simulink model "Model_Linearisierung_final"  (R2023b)
settings: Solver=FixedStepAuto  StartTime=0.0  StopTime=Inf  FixedStep=1e-4  RelTol=1e-3
PostLoadFcn:
  | if any(exist('dsrtsu_mdlpostloadfcn', 'file') ~= 0), dsrtsu_mdlpostloadfcn('Execute', bdroot); end
InitFcn:
  | , if any(exist('rtifpga_mdlclblib', 'file') ~= 0), rtifpga_mdlclblib('Init', bdroot); end,
  | , if any(exist('dsmpb_private', 'file') ~= 0), dsmpb_private('dsmpb_mdlclblib', 'Init', bdroot); end,
  | load('LUT_BRUSA_jax_grad.mat')
  | load('daten_nichtlinear_interpoliert.mat')
  | load('Maschinendaten.mat')
values from neighbouring files (symbols this model uses):
  delta_id = id_fine(2)-id_fine(1)    [Messdaten_Interpoliert.m]    (also in daten_nichtlinear_interpoliert.mat = 2.52525252525)
  delta_iq = iq_fine(2)-iq_fine(1)    [Messdaten_Interpoliert.m]    (also in daten_nichtlinear_interpoliert.mat = 5.05050505051)
  I_max = 170    [Maschinendaten.mat]    (also in Maschinendaten_Vorgabe.m; test_ModelParameters.m = evalin('base', 'I_max'); test_StrategySelection.m = tc.readConstant(tc.BLK_Imax))
  ID = [-250 -250 -250 -250 -250 -250 -250 -250 -250 -250 -250 -250 ... (10000 elements, 100x100)]    [daten_nichtlinear_interpoliert.mat]
  id_fine = linspace(min(id_vec), max(id_vec), 100)    [Messdaten_Interpoliert.m]    (also in daten_nichtlinear_interpoliert.mat = [-250 -247.474747475 -244.949494949 -242.424242424 -239.8989)
  IQ = [-250 -244.949494949 -239.898989899 -234.848484848 -229.797979798 -224.747474747 -219.696969697 -214.646464646 -209.595959596 -204.545454545 -199.494949495 -194.444444444 ... (10000 elements, 100x100)]    [daten_nichtlinear_interpoliert.mat]
  iq_fine = linspace(min(iq_vec), max(iq_vec), 100)    [Messdaten_Interpoliert.m]    (also in daten_nichtlinear_interpoliert.mat = [-250 -244.949494949 -239.898989899 -234.848484848 -229.7979)
  Ldd = Ldd_fine    [Messdaten_Interpoliert.m]    (also in daten_nichtlinear_interpoliert.mat = [0.000225276031415 0.000225750625371 0.000226241749969 0.000)
  Ldq = Ldq_fine    [Messdaten_Interpoliert.m]    (also in daten_nichtlinear_interpoliert.mat = [1.31113456519e-05 1.34236782585e-05 1.31001168558e-05 1.236)
  Lqd = Lqd_fine    [Messdaten_Interpoliert.m]    (also in daten_nichtlinear_interpoliert.mat = [7.22855329514e-05 7.00325573553e-05 6.7613098921e-05 6.5016)
  Lqq = Lqq_fine    [Messdaten_Interpoliert.m]    (also in daten_nichtlinear_interpoliert.mat = [0.000286039721686 0.000286453471045 0.000286025480511 0.000)
  n_max = 11000    [Maschinendaten.mat]    (also in Maschinendaten_Vorgabe.m; test_ModelParameters.m = evalin('base', 'n_max'); test_StrategySelection.m = tc.readConstant(tc.BLK_nmax))
  p = 3    [Maschinendaten.mat]    (also in Maschinendaten_Vorgabe.m; Messdaten_Interpoliert.m; test_ModelParameters.m = evalin('base', 'p'))
  Psid = Psid_fine    [Messdaten_Interpoliert.m]    (also in daten_nichtlinear_interpoliert.mat = [0.00602681114795 0.00609490588107 0.00615917040906 0.006219)
  Psiq = Psiq_fine    [Messdaten_Interpoliert.m]    (also in daten_nichtlinear_interpoliert.mat = [-0.166252688687 -0.164805403122 -0.163363500753 -0.16192610)
  Rs = 0.018    [Maschinendaten.mat]    (also in Maschinendaten_Vorgabe.m; test_ModelParameters.m = evalin('base', 'Rs'))
  U_dc = 560    [Maschinendaten.mat]    (also in Maschinendaten_Vorgabe.m; test_ModelParameters.m = evalin('base', 'U_dc'))
  U_max = 323.316150746    [Maschinendaten.mat]    (also in Maschinendaten_Vorgabe.m = U_dc / sqrt(3); test_ModelParameters.m = evalin('base', 'U_max'))
(part 1 of 3)
PreSaveFcn:
  | , if any(exist('dsmpb_private', 'file') ~= 0), dsmpb_private('dsmpb_mdlclblib', 'PreSave', bdroot); end,
CloseFcn:
  | , if any(exist('dsmpb_private', 'file') ~= 0), dsmpb_private('dsmpb_mdlclblib', 'Close', bdroot); end,
settings Model: DSRTSU_INTERNAL_RTIFPGA=210  DSRTSU_INTERNAL_RTISTBM_VER=24.2  DSMPB_ID_DATA={'1013',struct('BlockId','890db5c5-f774-4909-8d7b-80034ce0aceb','SignalIds',{{'dc619e18-1e49-4960-b686-3641b5b4e79b'}}),'722',struct('BlockId','8930e04f-7b9c-444e-9dfc-cdc89f8efc2c','SignalIds',{{'dce83508-d3d2-4435-9767-da790707202b'}}),'723',struct('BlockId','5d03b730-b193-419a-83cc-f730a6167e44','SignalIds',{{'20e4a8f8-d10b-4aad-9fba-86ba3280d00f'}}),'724',struct('BlockId','af5ca0db-6ef4-4fd1-9517-7edab6eec934','SignalIds',{{'0119e9a3-0335-4eef-8de2-1e0c5afd4a30'}})}  Creator=Student  LastModifiedBy=sarah
settings OptimizationCC: BlockReduction=off  ConditionallyExecuteInputs=off  OptimizeBlockIOStorage=off  BufferReuse=off
settings DebuggingCC: TasksWithSamePriorityMsg=none
settings HardwareCC: ProdBitPerLong=64  ProdLargestAtomicInteger=Integer  ProdWordSize=32  ProdLongLongMode=on  ProdHWDeviceType=Custom Processor->Custom
settings ModelReferenceCC: EnableParallelModelReferenceBuilds=on
settings RTWCC: Description=dSPACE Target DSRT - Generates SIC files for import by ConfigurationDesk and VEOS. Provides code generation for Simulink models imported in ConfigurationDesk.  SystemTargetFile=dsrt.tlc  GenCodeOnly=on  MakeCommand=make_dsrt  TemplateMakefile=dsrt_default_tmf  RTWVerbose=off
settings STFCustomTargetCC: ParMdlRefBuildCompliant=on  SystemTargetFile=dsrt.tlc
settings GRTTargetCC: CompOptLevelCompliant=off  ConcurrentExecutionCompliant=off  CombineOutputUpdateFcns=off  MatFileLogging=off  CPPClassGenCompliant=off  UseToolchainInfoCompliant=off

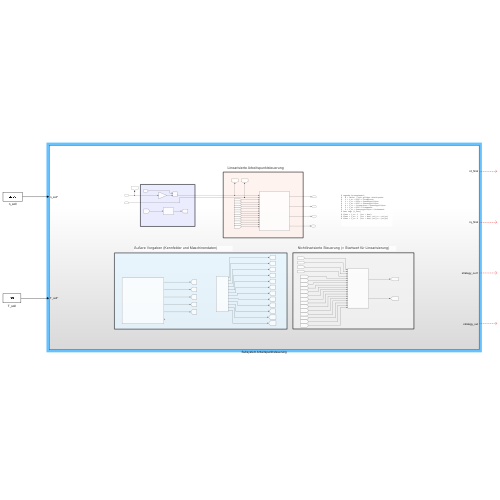
[thumbnail: Simulink's stored preview of the top-level diagram]
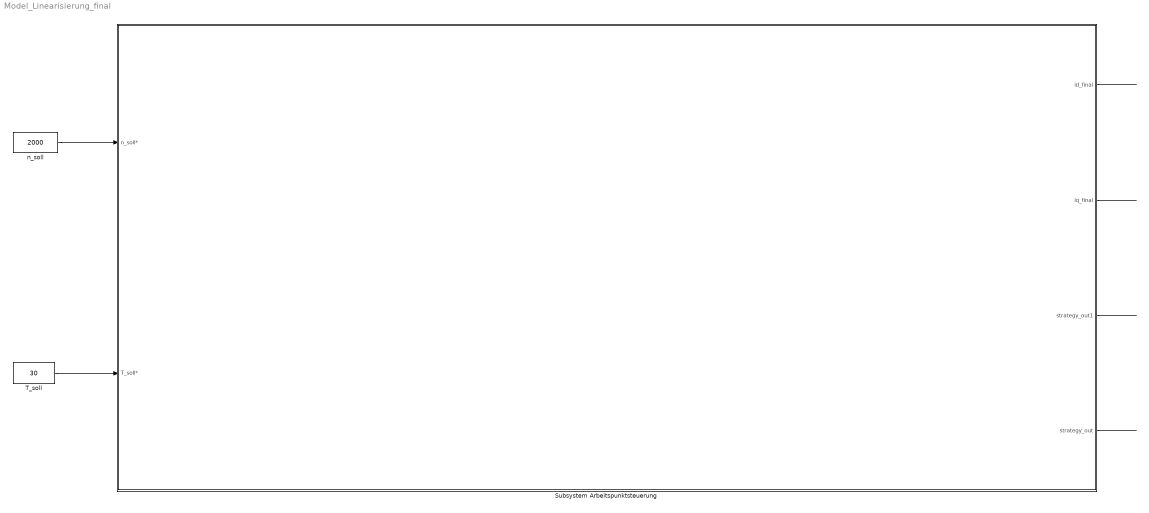
== system Model_Linearisierung_final ==
  Subsystem Arbeitspunktsteuerung : Subsystem
  T_soll : Constant  Value=30
  n_soll : Constant  Value=2000
  wires:
  n_soll/1 -> Subsystem Arbeitspunktsteuerung/1(n_soll*)
  T_soll/1 -> Subsystem Arbeitspunktsteuerung/2(T_soll*)
  Subsystem Arbeitspunktsteuerung/1(id_final) -> ?
  Subsystem Arbeitspunktsteuerung/2(iq_final) -> ?
  Subsystem Arbeitspunktsteuerung/4(strategy_out) -> ?
  Subsystem Arbeitspunktsteuerung/3(strategy_out1) -> ?

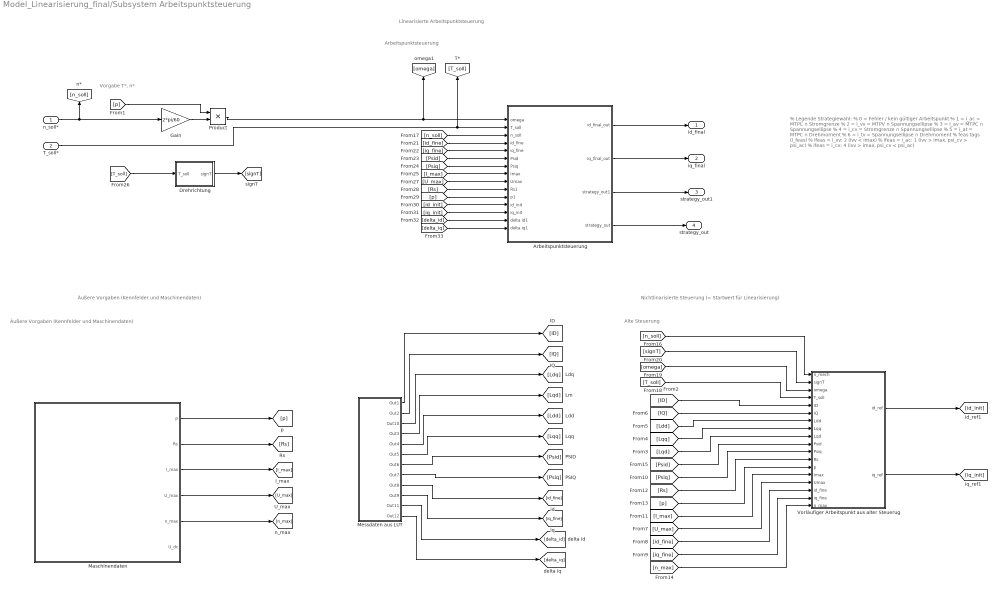
== system Model_Linearisierung_final/Subsystem Arbeitspunktsteuerung ==
  note: Vorgabe T*, n*
  note: % Legende Strategiewahl:
      | % 0 = Fehler / kein gültiger Arbeitspunkt
      | % 1 = i_ac = MTPC ∩ Stromgrenze
      | % 2 = i_vv = MTPV ∩ Spannungsellipse
      | % 3 = i_av = MTPC ∩ Spannungsellipse
      | % 4 = i_cv = Stromgrenze ∩ Spannungsellipse
      | % 5 = i_at = MTPC ∩ Drehmoment
      | % 6 = i_tv = Spannungsellipse ∩ Drehmoment
      | % feas tags (i_feas)
      | % ifeas = i_vv: 2 (ivv < imax)
      | % ifeas = i_ac: 1 (ivv > imax, psi_cv > psi_ac)
      | % ifeas = i_cv: 4 (ivv > imax, psi_cv < psi_ac)
  note: Nichtlinarisierte Steuerung (= Startwert für Linearisierung)
  note: Äußere Vorgaben (Kennfelder und Maschinendaten)
  note: Alte Steuerung
  note: Äußere Vorgaben (Kennfelder und Maschinendaten)
  note: Arbeitspunktsteuerung
  note: Linearisierte Arbeitspunktsteuerung
  n_soll* : Inport
  T_soll* : Inport  Port=2
  Arbeitspunktsteuerung : Subsystem
  Drehrichtung : MATLAB Function  Tag=<DSModel=2_'Model_Sarah'>  TreatAsAtomicUnit=on
      settings: AttributesFormatString=<DSModel='Model_Sarah'>
  Gain : Gain  Gain=2*pi/60
  Maschinendaten : Subsystem  Tag=<DSModel=5_'Model_Sarah'>
      settings: AttributesFormatString=<DSModel='Model_Sarah'>
  Messdaten aus LUT : Subsystem  Tag=<DSModel=4_'Model_Sarah'>
      settings: AttributesFormatString=<DSModel='Model_Sarah'>
  Product : Product
  Vorläufiger Arbeitspunkt aus alter Steuerug : Subsystem
  id_final : Outport
  iq_final : Outport  Port=2
  strategy_out1 : Outport  Port=3
  strategy_out : Outport  Port=4
  wires:
  Product/1 -> [omega], Arbeitspunktsteuerung/1(omega)
  Drehrichtung/1(signT) -> [signT]
  [n_soll] -> Arbeitspunktsteuerung/3(n_soll)
  Arbeitspunktsteuerung/2(iq_final_out) -> iq_final/1
  Arbeitspunktsteuerung/1(id_final_out) -> id_final/1
  T_soll*/1 -> [T_soll], Arbeitspunktsteuerung/2(T_soll)
  Arbeitspunktsteuerung/4(strategy_out) -> strategy_out/1
  [id_fine] -> Vorläufiger Arbeitspunkt aus alter Steuerug/16(id_fine)
  [Psid] -> Vorläufiger Arbeitspunkt aus alter Steuerug/10(Psid)
  Maschinendaten/5(n_max) -> [n_max]
  Maschinendaten/4(U_max) -> [U_max]
  Maschinendaten/1(" p") -> [p]
  Vorläufiger Arbeitspunkt aus alter Steuerug/1(id_ref) -> [id_init]
  [Ldd] -> Vorläufiger Arbeitspunkt aus alter Steuerug/7(Ldd)
  [Lqq] -> Vorläufiger Arbeitspunkt aus alter Steuerug/8(Lqq)
  Messdaten aus LUT/6(Out5) -> [Lqq]
  Vorläufiger Arbeitspunkt aus alter Steuerug/2(iq_ref) -> [iq_init]
  [T_soll] -> Vorläufiger Arbeitspunkt aus alter Steuerug/4(T_soll)
  Maschinendaten/3(" I_max") -> [I_max]
  Messdaten aus LUT/8(Out7) -> [Psiq]
  [U_max] -> Vorläufiger Arbeitspunkt aus alter Steuerug/15(Umax)
  [Lqd] -> Vorläufiger Arbeitspunkt aus alter Steuerug/9(Lqd)
  [Rs] -> Vorläufiger Arbeitspunkt aus alter Steuerug/12(Rs)
  [n_max] -> Vorläufiger Arbeitspunkt aus alter Steuerug/18(n_max)
  [p] -> Vorläufiger Arbeitspunkt aus alter Steuerug/13(p)
  [Psiq] -> Vorläufiger Arbeitspunkt aus alter Steuerug/11(Psiq)
  [IQ] -> Vorläufiger Arbeitspunkt aus alter Steuerug/6(IQ)
  [ID] -> Vorläufiger Arbeitspunkt aus alter Steuerug/5(ID)
  [n_soll] -> Vorläufiger Arbeitspunkt aus alter Steuerug/1(n_mech)
  [iq_fine] -> Vorläufiger Arbeitspunkt aus alter Steuerug/17(iq_fine)
  [I_max] -> Vorläufiger Arbeitspunkt aus alter Steuerug/14(Imax)
  Messdaten aus LUT/5(Out4) -> [Ldd]
  Messdaten aus LUT/2(Out2) -> [IQ]
  Messdaten aus LUT/4(Out3) -> [Lqd]
  [omega] -> Vorläufiger Arbeitspunkt aus alter Steuerug/3(omega)
  Messdaten aus LUT/10(Out9) -> [iq_fine]
  Messdaten aus LUT/11(Out11) -> [delta_id]
  Messdaten aus LUT/7(Out6) -> [Psid]
  Messdaten aus LUT/3(Out10) -> [Ldq]
  Maschinendaten/2(" Rs") -> [Rs]
  Messdaten aus LUT/12(Out12) -> [delta_iq]
  Messdaten aus LUT/9(Out8) -> [id_fine]
  Messdaten aus LUT/1(Out1) -> [ID]
  [T_soll] -> Drehrichtung/1(T_soll)
  n_soll*/1 -> Gain/1, [n_soll]
  Gain/1 -> Product/2
  [p] -> Product/1
  [signT] -> Vorläufiger Arbeitspunkt aus alter Steuerug/2(signT)
  [id_fine] -> Arbeitspunktsteuerung/4(id_fine)
  [iq_fine] -> Arbeitspunktsteuerung/5(iq_fine)
  [Psid] -> Arbeitspunktsteuerung/6(Psid)
  [Psiq] -> Arbeitspunktsteuerung/7(Psiq)
  [I_max] -> Arbeitspunktsteuerung/8(Imax)
  [p] -> Arbeitspunktsteuerung/11(p1)
  [Rs] -> Arbeitspunktsteuerung/10(Rs1)
  [U_max] -> Arbeitspunktsteuerung/9(Umax)
  [id_init] -> Arbeitspunktsteuerung/12(id_init)
  [iq_init] -> Arbeitspunktsteuerung/13(iq_init)
  [delta_id] -> Arbeitspunktsteuerung/14(delta id1)
  [delta_iq] -> Arbeitspunktsteuerung/15(delta iq1)
  Arbeitspunktsteuerung/3(strategy_out1) -> strategy_out1/1

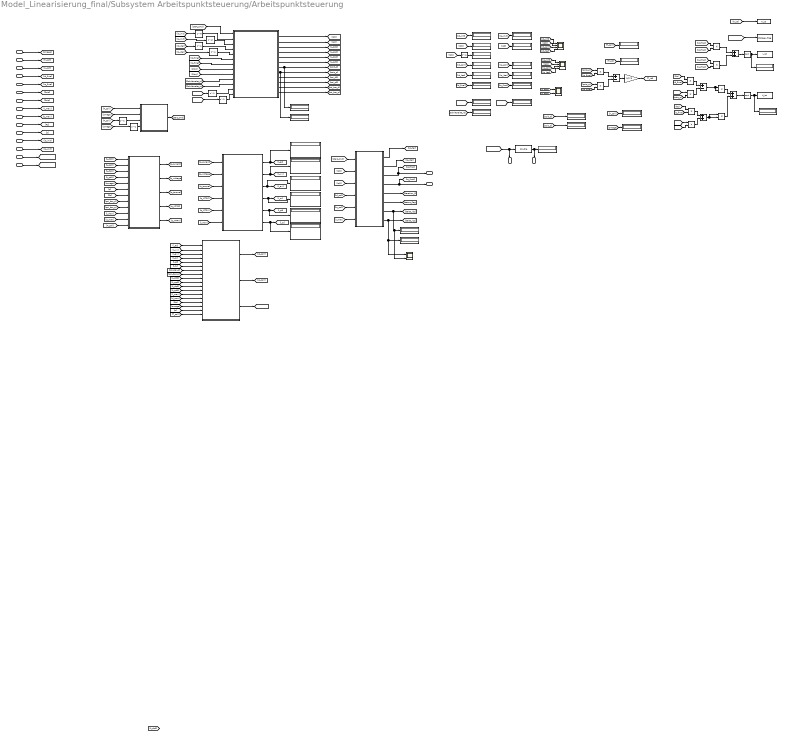
== system Model_Linearisierung_final/Subsystem Arbeitspunktsteuerung/Arbeitspunktsteuerung ==
  note: Neue Regelung
  note: % Legende Strategiewahl:
      | % 0 = Fehler / kein gültiger Arbeitspunkt
      | % 1 = i_ac = MTPC ∩ Stromgrenze
      | % 2 = i_vv = MTPV ∩ Spannungsellipse
      | % 3 = i_av = MTPC ∩ Spannungsellipse
      | % 4 = i_cv = Stromgrenze ∩ Spannungsellipse
      | % 5 = i_at = MTPC ∩ Drehmoment
      | % 6 = i_tv = Spannungsellipse ∩ Drehmoment
      | % feas tags (i_feas)
      | % ifeas = i_vv: 2 (ivv < imax)
      | % ifeas = i_ac: 1 (ivv > imax, psi_cv > psi_ac)
      | % ifeas = i_cv: 4 (ivv > imax, psi_cv < psi_ac)
  note: Überwachung
  note: Regelung mit Linearisierung um den Arbeitspunkt
  note: Überwachung der Werte
  note: Ströme
  note: Strategiewahl
  note: Drehmoment
  note: Drehzahl
  note: Induktivitäten
  note: Alte Regelung
  note: Äußere Eingänge
  note: Überwachung
  note: Ausgabe der Werte für Github
  note: U_ist = sqrt(ud^2 + uq^2)
      |
      | ud = Rs*id_final - omega*psiq
      | uq = Rs*iq_final + omega*psid
  note: Ausgabe Drehmoment
  note: Ausgabe Strategie
  note: Ausgabe Strom
  note: Ausgabe Spannung
  omega : Inport
  T_soll : Inport  Port=2
  n_soll : Inport  Port=3
  id_fine : Inport  Port=4
  iq_fine : Inport  Port=5
  Psid : Inport  Port=6
  Psiq : Inport  Port=7
  Imax : Inport  Port=8
  Umax : Inport  Port=9
  Rs1 : Inport  Port=10
  p1 : Inport  Port=11
  id_init : Inport  Port=12
  iq_init : Inport  Port=13
  delta id1 : Inport  Port=14
  delta iq1 : Inport  Port=15
  Ausgabe I_ist1 : Display
  Ausgabe Strategiewahl : Display
  Ausgabe T_ist : Display
  Ausgabe U_ist1 : Display
  Ausgabe omega : Display
  Data Type Conversion : DataTypeConversion  OutDataTypeStr=double  SaturateOnIntegerOverflow=off  RndMeth=Floor
  Delay : Delay  DelayLength=0
  Delay1 : Delay  DelayLength=0
  Delay{2..8} (7 alike) : Delay  DelayLength=1
  Delta id : Display
  Glac - Arbeitspunktwahl : MATLAB Function  TreatAsAtomicUnit=on
  Glac - Schnittpunktsuche : MATLAB Function  TreatAsAtomicUnit=on
  Induktivitäten L : Scope  NumInputPorts=2
  Induktivitäten L1 : Scope  NumInputPorts=2
  Iterationsblock : MATLAB Function  TreatAsAtomicUnit=on
  Iterationsschritt : Display
  Linearisierung um idq0 : MATLAB Function  TreatAsAtomicUnit=on
  Multiply : Gain  Gain=3/2*3
  Product{,1..9} (10 alike) : Product
  Quadriken Hackl : MATLAB Function  TreatAsAtomicUnit=on
  Sqrt : Sqrt
  Sqrt1 : Sqrt
  Startflanke für Berechnung : MATLAB Function  TreatAsAtomicUnit=on
  Startimpuls : Display
  Subtract : Sum  Inputs=+-
  Subtract1 : Sum
  Subtract2 : Sum
  Subtract3 : Sum  Inputs=+-
  Subtract4 : Sum
  To Workspace1 : ToWorkspace  VariableName=T_ist  SaveFormat=Timeseries  SampleTime=-1
  To Workspace2 : ToWorkspace  VariableName=strategy_flag  SaveFormat=Timeseries  SampleTime=-1
  To Workspace3 : ToWorkspace  VariableName=I_ist  SaveFormat=Timeseries  SampleTime=-1
  To Workspace4 : ToWorkspace  VariableName=U_ist  SaveFormat=Timeseries  SampleTime=-1
  Vergleich iq : Scope  NumInputPorts=4
  Verleich id : Scope  NumInputPorts=4
  Vorgabe T_soll : Display
  Vorgabe id0 : Display
  Vorgabe id1 : Display
  Vorgabe id_final1 : Display
  Vorgabe id_iter1 : Display
  Vorgabe id_ref1 : Display
  Vorgabe id_soll1 : Display
  Vorgabe iq0 : Display
  Vorgabe iq_final1 : Display
  Vorgabe iq_iter1 : Display
  Vorgabe iq_ref1 : Display
  Vorgabe iq_soll1 : Display
  Vorgabe n_soll1 : Display
  i_ac : Display
  i_at : Display
  i_av : Display
  i_cv : Display
  i_tv : Display
  i_vv : Display
  psid1 : Display
  psid2 : Display
  psid_0 : Display
  psiq1 : Display
  psiq2 : Display
  psiq_0 : Display
  id_final_out : Outport
  iq_final_out : Outport  Port=2
  strategy_out1 : Outport  Port=3
  strategy_out : Outport  Port=4
  wires:
  Linearisierung um idq0/1(id0_out) -> [id0]
  Linearisierung um idq0/2(iq0_out) -> [iq0]
  Linearisierung um idq0/3(L_dd0) -> [L_dd0]
  Linearisierung um idq0/4(L_qq0) -> [L_qq0]
  [id_soll] -> Iterationsblock/4(id_soll)
  [iq_soll] -> Iterationsblock/5(iq_soll)
  [id0] -> Iterationsblock/2(id0)
  [iq0] -> Iterationsblock/3(iq0)
  Delay/1 -> Linearisierung um idq0/2(id_init)
  Delay1/1 -> Linearisierung um idq0/3(iq_init)
  Iterationsblock/1(id_iter) -> [id_iter]
  Iterationsblock/2(iq_iter) -> [iq_iter]
  Iterationsblock/3(id_final) -> [id_final], id_final_out/1
  Iterationsblock/4(iq_final) -> [iq_final], iq_final_out/1
  Iterationsblock/5(iter_count) -> [Iteration_k]
  Iterationsblock/6(status_flag) -> [status_flag]
  [I_max] -> Iterationsblock/6(I_max)
  Startflanke für Berechnung/1(start_cmd) -> [start_cmd]
  Delay3/1 -> Startflanke für Berechnung/4(omega_z1)
  [omega] -> Delay3/1
  Delay2/1 -> Startflanke für Berechnung/3(T_soll_z1)
  [T_soll] -> Delay2/1
  [T_soll] -> Startflanke für Berechnung/1(T_soll)
  [omega] -> Startflanke für Berechnung/2(omega)
  [start_cmd] -> Iterationsblock/1(start_cmd)
  [start_cmd] -> Linearisierung um idq0/1(start_cmd)
  Delay5/1 -> Linearisierung um idq0/5(iq_iter)
  [iq_iter] -> Delay5/1
  Delay4/1 -> Linearisierung um idq0/4(id_iter)
  [id_iter] -> Delay4/1
  [id_init] -> Vorgabe id_ref1/1
  [id_final] -> Vorgabe id_final1/1
  [id_iter] -> Vorgabe id_iter1/1
  [id_soll] -> Vorgabe id_soll1/1
  [id0] -> Vorgabe id0/1
  [iq_init] -> Vorgabe iq_ref1/1
  [iq0] -> Vorgabe iq0/1
  [iq_soll] -> Vorgabe iq_soll1/1
  [iq_iter] -> Vorgabe iq_iter1/1
  [iq_final] -> Vorgabe iq_final1/1
  [id0] -> Delay6/1
  Delay6/1 -> Vorgabe id1/1
  [start_cmd] -> Startimpuls/1
  [Schrittweite_id] -> Delta id/1
  Glac - Schnittpunktsuche/1(i_ac) -> i_ac/1, [i_ac]
  [id_init] -> Verleich id/1
  [id0] -> Verleich id/2
  [id_soll] -> Verleich id/3
  [id_iter] -> Verleich id/4
  [iq_init] -> Vergleich iq/1
  [iq_soll] -> Vergleich iq/3
  [iq0] -> Vergleich iq/2
  [iq_iter] -> Vergleich iq/4
  [L_qq0] -> Induktivitäten L/2
  [L_dd0] -> Induktivitäten L/1
  [Iteration_k] -> Iterationsschritt/1
  [T_soll] -> Vorgabe T_soll/1
  [T_ist] -> Ausgabe T_ist/1
  [psid_d] -> Product/1
  [iq_final] -> Product/2
  [id_final] -> Product1/2
  [psiq_q] -> Product1/1
  Product/1 -> Subtract/1
  Product1/1 -> Subtract/2
  Subtract/1 -> Multiply/1
  Multiply/1 -> [T_ist]
  [n_soll] -> Vorgabe n_soll1/1
  [omega] -> Ausgabe omega/1
  [strategy_flag] -> strategy_out1/1, Data Type Conversion/1
  Data Type Conversion/1 -> strategy_out/1, Ausgabe Strategiewahl/1
  [psid_d] -> psid_0/1
  [psiq_q] -> psiq_0/1
  Iterationsblock/7(delta_id) -> Induktivitäten L1/2, psid2/1, [delta_id1]
  Iterationsblock/8(delta_iq) -> Induktivitäten L1/1, psiq2/1, [delta_iq1]
  [Schrittweite_id] -> Linearisierung um idq0/10(Schrittweite_id)
  [Schrittweite_iq] -> Linearisierung um idq0/11(Schrittweite_iq)
  [delta_id1] -> Delay8/1
  [delta_iq1] -> Delay7/1
  Delay7/1 -> Linearisierung um idq0/13(delta_iq_last)
  Delay8/1 -> Linearisierung um idq0/12(delta_id_last)
  Linearisierung um idq0/7(psid_d) -> psid1/1, [psid_d]
  Linearisierung um idq0/8(psiq_q) -> psiq1/1, [psiq_q]
  Linearisierung um idq0/5(L_dq0) -> [L_dq0]
  [U_max] -> Glac - Arbeitspunktwahl/14(Umax)
  [p] -> Quadriken Hackl/6(p)
  [Rs] -> Quadriken Hackl/7(Rs)
  [omega] -> Quadriken Hackl/5(omega)
  [L_qq0] -> Quadriken Hackl/2(Lqq)
  [I_max] -> Quadriken Hackl/10(Imax)
  [L_dq0] -> Quadriken Hackl/3(Ldq)
  [L_dd0] -> Quadriken Hackl/1(Ldd)
  [U_max] -> Quadriken Hackl/11(Umax)
  [q_MTPC] -> Glac - Schnittpunktsuche/4(q_MTPC)
  [q_MTPV] -> Glac - Schnittpunktsuche/5(q_MTPV)
  Glac - Schnittpunktsuche/3(i_av) -> i_av/1, [i_av]
  Glac - Schnittpunktsuche/5(i_at) -> i_at/1, [i_at]
  Glac - Schnittpunktsuche/6(i_tv) -> i_tv/1, [i_tv]
  [I_max] -> Glac - Arbeitspunktwahl/13(Imax)
  [T_soll] -> Glac - Arbeitspunktwahl/18(T_soll)
  [i_tv] -> Glac - Arbeitspunktwahl/6(i_tv)
  [i_at] -> Glac - Arbeitspunktwahl/5(i_at)
  [i_cv] -> Glac - Arbeitspunktwahl/4(i_cv)
  [i_av] -> Glac - Arbeitspunktwahl/3(i_av)
  [i_vv] -> Glac - Arbeitspunktwahl/2(i_vv)
  [i_ac] -> Glac - Arbeitspunktwahl/1(i_ac)
  Glac - Arbeitspunktwahl/1(id_soll) -> [id_soll]
  Glac - Arbeitspunktwahl/2(iq_soll) -> [iq_soll]
  Linearisierung um idq0/9(psi_d0) -> [psi_d0]
  Linearisierung um idq0/10(psi_q0) -> [psi_q0]
  [psi_bar_d] -> Glac - Arbeitspunktwahl/7(psi_bar_d)
  [psi_bar_q] -> Glac - Arbeitspunktwahl/8(psi_bar_q)
  [L_dd0] -> Glac - Arbeitspunktwahl/9(Ldd)
  [L_qq0] -> Glac - Arbeitspunktwahl/10(Lqq)
  [L_dq0] -> Glac - Arbeitspunktwahl/11(Ldq)
  [I_max] -> Glac - Schnittpunktsuche/6(Imax)
  Glac - Schnittpunktsuche/2(i_vv) -> i_vv/1, [i_vv]
  Glac - Arbeitspunktwahl/3(strategy_flag) -> [strategy_flag]
  Linearisierung um idq0/6(L_qd0) -> [L_qd0]
  [L_qd0] -> Quadriken Hackl/4(Lqd)
  Linearisierung um idq0/11(psi_bar_d) -> [psi_bar_d]
  Linearisierung um idq0/12(psi_bar_q) -> [psi_bar_q]
  [psi_bar_d] -> Quadriken Hackl/8(psi_bar_d)
  [psi_bar_q] -> Quadriken Hackl/9(psi_bar_q)
  [T_soll] -> Quadriken Hackl/12(T_soll)
  Quadriken Hackl/5(q_MTPV) -> [q_MTPV]
  Quadriken Hackl/2(q_voltage) -> [q_voltage]
  Quadriken Hackl/3(q_torque) -> [q_torque]
  Quadriken Hackl/4(q_MTPC) -> [q_MTPC]
  Quadriken Hackl/1(q_current) -> [q_current]
  [q_torque] -> Glac - Schnittpunktsuche/3(q_torque)
  [q_voltage] -> Glac - Schnittpunktsuche/2(q_voltage)
  [q_current] -> Glac - Schnittpunktsuche/1(q_current)
  [Rs] -> Glac - Arbeitspunktwahl/15(Rs)
  [omega] -> Glac - Arbeitspunktwahl/16(omega)
  [p] -> Glac - Arbeitspunktwahl/17(p)
  [L_qd0] -> Glac - Arbeitspunktwahl/12(Lqd)
  Glac - Schnittpunktsuche/4(i_cv) -> [i_cv], i_cv/1
  [Psid] -> Linearisierung um idq0/8(Psid)
  [Psiq] -> Linearisierung um idq0/9(Psiq)
  [iq_fine] -> Linearisierung um idq0/7(iq_fine)
  [id_fine] -> Linearisierung um idq0/6(id_fine)
  [id_init] -> Delay/1
  [iq_init] -> Delay1/1
  omega/1 -> [omega]
  T_soll/1 -> [T_soll]
  n_soll/1 -> [n_soll]
  id_fine/1 -> [id_fine]
  iq_fine/1 -> [iq_fine]
  Psid/1 -> [Psid]
  Psiq/1 -> [Psiq]
  Imax/1 -> [I_max]
  Umax/1 -> [U_max]
  Rs1/1 -> [Rs]
  id_init/1 -> [id_init]
  iq_init/1 -> [iq_init]
  delta id1/1 -> [Schrittweite_id]
  delta iq1/1 -> [Schrittweite_iq]
  p1/1 -> [p]
  [T_ist] -> To Workspace1/1
  [strategy_flag] -> To Workspace2/1
  [id_final] -> Product2/1
  [id_final] -> Product2/2
  [iq_final] -> Product3/1
  Product3/1 -> Subtract1/2
  Product2/1 -> Subtract1/1
  Subtract1/1 -> Sqrt/1
  Sqrt/1 -> Ausgabe I_ist1/1, To Workspace3/1
  [iq_final] -> Product3/2
  Subtract2/1 -> Sqrt1/1
  Sqrt1/1 -> Ausgabe U_ist1/1, To Workspace4/1
  [Rs] -> Product6/1
  [id_final] -> Product6/2
  Product6/1 -> Subtract3/1
  [omega] -> Product7/1
  Product7/1 -> Subtract3/2
  [psid_d] -> Product8/2
  Product8/1 -> Subtract4/2
  [Rs] -> Product4/1
  [iq_final] -> Product4/2
  [omega] -> Product8/1
  Product4/1 -> Subtract4/1
  [psiq_q] -> Product7/2
  Subtract3/1 -> Product9/2, Product9/1
  Subtract4/1 -> Product5/2, Product5/1
  Product5/1 -> Subtract2/2
  Product9/1 -> Subtract2/1

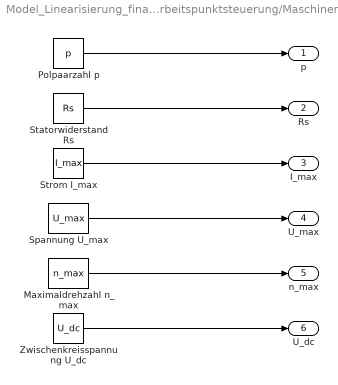
== system Model_Linearisierung_final/Subsystem Arbeitspunktsteuerung/Maschinendaten ==
  Maximaldrehzahl n_max : Constant  Value=n_max
  Polpaarzahl p : Constant  Value=p
  Spannung U_max : Constant  Value=U_max
  Statorwiderstand Rs : Constant  Value=Rs
  Strom I_max : Constant  Value=I_max
  Zwischenkreisspannung U_dc : Constant  Value=U_dc
  " p" : Outport
  " Rs" : Outport  Port=2
  " I_max" : Outport  Port=3
  U_max : Outport  Port=4
  n_max : Outport  Port=5
  " U_dc" : Outport  Port=6
  wires:
  Maximaldrehzahl n_max/1 -> n_max/1
  Spannung U_max/1 -> U_max/1
  Statorwiderstand Rs/1 -> " Rs"/1
  Polpaarzahl p/1 -> " p"/1
  Strom I_max/1 -> " I_max"/1
  Zwischenkreisspannung U_dc/1 -> " U_dc"/1

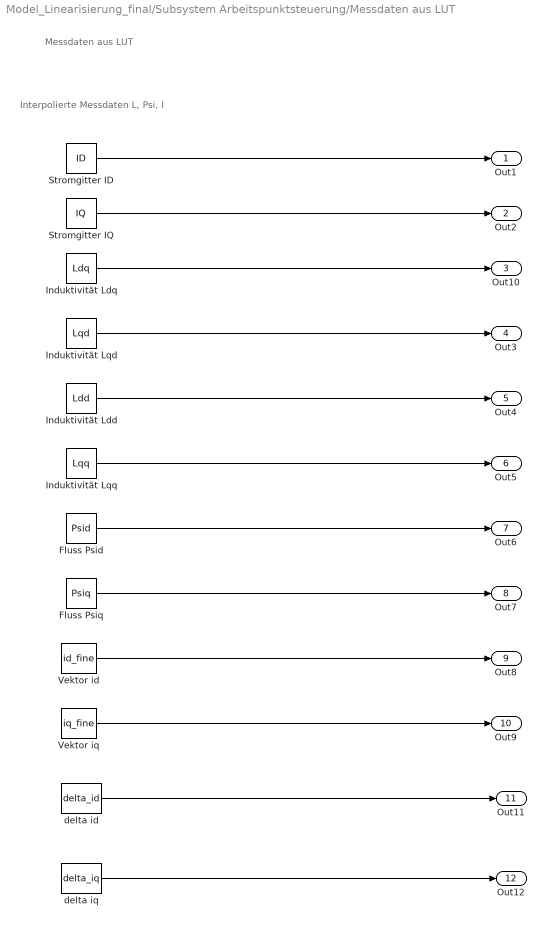
== system Model_Linearisierung_final/Subsystem Arbeitspunktsteuerung/Messdaten aus LUT ==
  note: Messdaten aus LUT
  note: Interpolierte Messdaten L, Psi, I
  Fluss Psid : Constant  Value=Psid
  Fluss Psiq : Constant  Value=Psiq
  Induktivität Ldd : Constant  Value=Ldd
  Induktivität Ldq : Constant  Value=Ldq
  Induktivität Lqd : Constant  Value=Lqd
  Induktivität Lqq : Constant  Value=Lqq
  Stromgitter ID : Constant  Value=ID
  Stromgitter IQ : Constant  Value=IQ
  Vektor id : Constant  Value=id_fine
  Vektor iq : Constant  Value=iq_fine
  delta id : Constant  Value=delta_id
  delta iq : Constant  Value=delta_iq
  Out1 : Outport
  Out2 : Outport  Port=2
  Out10 : Outport  Port=3
  Out3 : Outport  Port=4
  Out4 : Outport  Port=5
  Out5 : Outport  Port=6
  Out6 : Outport  Port=7
  Out7 : Outport  Port=8
  Out8 : Outport  Port=9
  Out9 : Outport  Port=10
  Out11 : Outport  Port=11
  Out12 : Outport  Port=12
  wires:
  Vektor id/1 -> Out8/1
  Vektor iq/1 -> Out9/1
  Stromgitter ID/1 -> Out1/1
  Stromgitter IQ/1 -> Out2/1
  Fluss Psid/1 -> Out6/1
  Fluss Psiq/1 -> Out7/1
  Induktivität Lqd/1 -> Out3/1
  Induktivität Ldd/1 -> Out4/1
  Induktivität Lqq/1 -> Out5/1
  Induktivität Ldq/1 -> Out10/1
  delta id/1 -> Out11/1
  delta iq/1 -> Out12/1

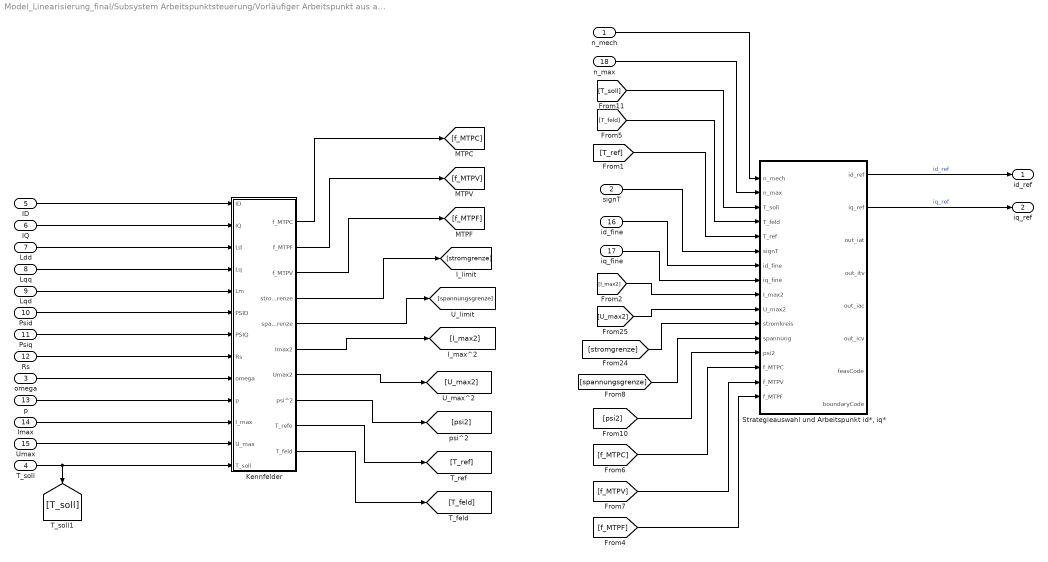
== system Model_Linearisierung_final/Subsystem Arbeitspunktsteuerung/Vorläufiger Arbeitspunkt aus alter Steuerug ==
  n_mech : Inport
  signT : Inport  Port=2
  omega : Inport  Port=3
  T_soll : Inport  Port=4
  ID : Inport  Port=5
  IQ : Inport  Port=6
  Ldd : Inport  Port=7
  Lqq : Inport  Port=8
  Lqd : Inport  Port=9
  Psid : Inport  Port=10
  Psiq : Inport  Port=11
  Rs : Inport  Port=12
  p : Inport  Port=13
  Imax : Inport  Port=14
  Umax : Inport  Port=15
  id_fine : Inport  Port=16
  iq_fine : Inport  Port=17
  n_max : Inport  Port=18
  Kennfelder : Subsystem  Tag=<DSModel=3_'Model_Sarah'>
      settings: AttributesFormatString=<DSModel='Model_Sarah'>
  "Strategieauswahl und Arbeitspunkt id*, iq*" : MATLAB Function  Tag=<DSModel=1_'Model_Sarah'>  TreatAsAtomicUnit=on
      settings: AttributesFormatString=<DSModel='Model_Sarah'>
  id_ref : Outport
  iq_ref : Outport  Port=2
  wires:
  [spannungsgrenze] -> "Strategieauswahl und Arbeitspunkt id*, iq*"/12(spannung)
  Kennfelder/3(f_MTPV) -> [f_MTPF]
  Umax/1 -> Kennfelder/12(U_max)
  Lqd/1 -> Kennfelder/5(Lm)
  Psiq/1 -> Kennfelder/7(PSIQ)
  signT/1 -> "Strategieauswahl und Arbeitspunkt id*, iq*"/6(signT)
  Rs/1 -> Kennfelder/8(Rs)
  p/1 -> Kennfelder/10(p)
  [I_max2] -> "Strategieauswahl und Arbeitspunkt id*, iq*"/9(I_max2)
  omega/1 -> Kennfelder/9(omega)
  Kennfelder/7(Umax2) -> [U_max2]
  [T_soll] -> "Strategieauswahl und Arbeitspunkt id*, iq*"/3(T_soll)
  ID/1 -> Kennfelder/1(ID)
  [f_MTPF] -> "Strategieauswahl und Arbeitspunkt id*, iq*"/16(f_MTPF)
  [T_ref] -> "Strategieauswahl und Arbeitspunkt id*, iq*"/5(T_ref)
  Kennfelder/2(f_MTPF) -> [f_MTPV]
  Kennfelder/5(spannungsgrenze) -> [spannungsgrenze]
  iq_fine/1 -> "Strategieauswahl und Arbeitspunkt id*, iq*"/8(iq_fine)
  Kennfelder/9(T_refe) -> [T_ref]
  [f_MTPC] -> "Strategieauswahl und Arbeitspunkt id*, iq*"/14(f_MTPC)
  Psid/1 -> Kennfelder/6(PSID)
  [psi2] -> "Strategieauswahl und Arbeitspunkt id*, iq*"/13(psi2)
  Kennfelder/8(psi^2) -> [psi2]
  [T_feld] -> "Strategieauswahl und Arbeitspunkt id*, iq*"/4(T_feld)
  Ldd/1 -> Kennfelder/3(Ld)
  [U_max2] -> "Strategieauswahl und Arbeitspunkt id*, iq*"/10(U_max2)
  T_soll/1 -> [T_soll], Kennfelder/13(T_soll)
  [stromgrenze] -> "Strategieauswahl und Arbeitspunkt id*, iq*"/11(stromkreis)
  Kennfelder/4(stromgrenze) -> [stromgrenze]
  n_max/1 -> "Strategieauswahl und Arbeitspunkt id*, iq*"/2(n_max)
  Kennfelder/10(T_feld) -> [T_feld]
  [f_MTPV] -> "Strategieauswahl und Arbeitspunkt id*, iq*"/15(f_MTPV)
  IQ/1 -> Kennfelder/2(IQ)
  Kennfelder/1(f_MTPC) -> [f_MTPC]
  "Strategieauswahl und Arbeitspunkt id*, iq*"/1(id_ref) -> id_ref/1  "id_ref"
  n_mech/1 -> "Strategieauswahl und Arbeitspunkt id*, iq*"/1(n_mech)
  id_fine/1 -> "Strategieauswahl und Arbeitspunkt id*, iq*"/7(id_fine)
  Imax/1 -> Kennfelder/11(I_max)
  Kennfelder/6(Imax2) -> [I_max2]
  Lqq/1 -> Kennfelder/4(Lq)
  "Strategieauswahl und Arbeitspunkt id*, iq*"/2(iq_ref) -> iq_ref/1  "iq_ref"

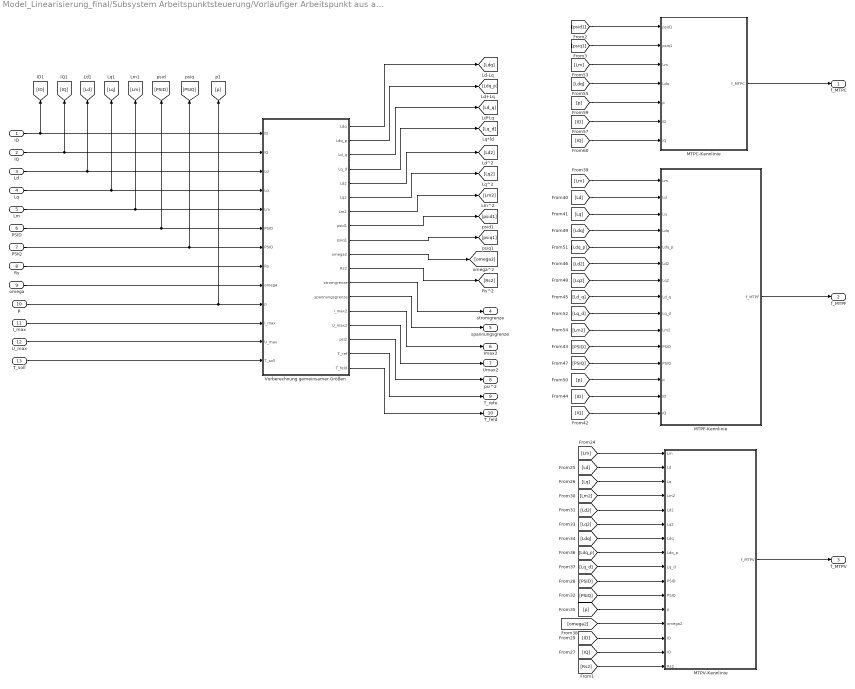
== system Model_Linearisierung_final/Subsystem Arbeitspunktsteuerung/Vorläufiger Arbeitspunkt aus alter Steuerug/Kennfelder ==
  ID : Inport
  IQ : Inport  Port=2
  Ld : Inport  Port=3
  Lq : Inport  Port=4
  Lm : Inport  Port=5
  PSID : Inport  Port=6
  PSIQ : Inport  Port=7
  Rs : Inport  Port=8
  omega : Inport  Port=9
  p : Inport  Port=10
  I_max : Inport  Port=11
  U_max : Inport  Port=12
  T_soll : Inport  Port=13
  " Vorberechnung gemeinsamer Größen" : MATLAB Function  TreatAsAtomicUnit=on
  MTPC-Kennlinie : MATLAB Function  TreatAsAtomicUnit=on
  MTPF-Kennlinie : MATLAB Function  TreatAsAtomicUnit=on
  MTPV-Kennlinie : MATLAB Function  TreatAsAtomicUnit=on
  f_MTPC : Outport
  f_MTPF : Outport  Port=2
  f_MTPV : Outport  Port=3
  stromgrenze : Outport  Port=4
  spannungsgrenze : Outport  Port=5
  Imax2 : Outport  Port=6
  Umax2 : Outport  Port=7
  psi^2 : Outport  Port=8
  T_refe : Outport  Port=9
  T_feld : Outport  Port=10
  wires:
  T_soll/1 -> " Vorberechnung gemeinsamer Größen"/13(T_soll)
  " Vorberechnung gemeinsamer Größen"/18(T_feld) -> T_feld/1
  " Vorberechnung gemeinsamer Größen"/17(T_ref) -> T_refe/1
  " Vorberechnung gemeinsamer Größen"/16(psi2) -> psi^2/1
  " Vorberechnung gemeinsamer Größen"/14(I_max2) -> Imax2/1
  " Vorberechnung gemeinsamer Größen"/15(U_max2) -> Umax2/1
  [Rs2] -> MTPV-Kennlinie/16(Rs2)
  MTPV-Kennlinie/1(f_MTPV) -> f_MTPV/1
  MTPC-Kennlinie/1(f_MTPC) -> f_MTPC/1
  MTPF-Kennlinie/1(f_MTPF) -> f_MTPF/1
  PSID/1 -> " Vorberechnung gemeinsamer Größen"/6(PSID), [PSID]
  Lm/1 -> " Vorberechnung gemeinsamer Größen"/5(Lm), [Lm]
  U_max/1 -> " Vorberechnung gemeinsamer Größen"/12(U_max)
  Lq/1 -> " Vorberechnung gemeinsamer Größen"/4(Lq), [Lq]
  I_max/1 -> " Vorberechnung gemeinsamer Größen"/11(I_max)
  IQ/1 -> " Vorberechnung gemeinsamer Größen"/2(IQ), [IQ]
  p/1 -> " Vorberechnung gemeinsamer Größen"/10(p), [p]
  PSIQ/1 -> " Vorberechnung gemeinsamer Größen"/7(PSIQ), [PSIQ]
  [Ldq] -> MTPF-Kennlinie/4(Ldq)
  [omega2] -> MTPV-Kennlinie/13(omega2)
  omega/1 -> " Vorberechnung gemeinsamer Größen"/9(omega)
  [Ld2] -> MTPF-Kennlinie/6(Ld2)
  [Lq] -> MTPV-Kennlinie/3(Lq)
  [Lm] -> MTPV-Kennlinie/1(Lm)
  " Vorberechnung gemeinsamer Größen"/7(Lm2) -> [Lm2]
  [Ld] -> MTPF-Kennlinie/2(Ld)
  [Ldq_p] -> MTPV-Kennlinie/8(Ldq_p)
  [Ldq] -> MTPV-Kennlinie/7(Ldq)
  " Vorberechnung gemeinsamer Größen"/3(Ld_q) -> [Ld_q]
  [Lq2] -> MTPV-Kennlinie/6(Lq2)
  [ID] -> MTPV-Kennlinie/14(ID)
  [PSIQ] -> MTPF-Kennlinie/12(PSIQ)
  " Vorberechnung gemeinsamer Größen"/4(Lq_d) -> [Lq_d]
  [p] -> MTPC-Kennlinie/5(p)
  " Vorberechnung gemeinsamer Größen"/8(psid1) -> [psid1]
  [Lq_d] -> MTPV-Kennlinie/9(Lq_d)
  Ld/1 -> " Vorberechnung gemeinsamer Größen"/3(Ld), [Ld]
  [ID] -> MTPF-Kennlinie/14(ID)
  Rs/1 -> " Vorberechnung gemeinsamer Größen"/8(Rs)
  " Vorberechnung gemeinsamer Größen"/1(Ldq) -> [Ldq]
  [Ldq_p] -> MTPF-Kennlinie/5(Ldq_p)
  [IQ] -> MTPV-Kennlinie/15(IQ)
  [PSID] -> MTPV-Kennlinie/10(PSID)
  " Vorberechnung gemeinsamer Größen"/10(omega2) -> [omega2]
  " Vorberechnung gemeinsamer Größen"/13(spannungsgrenze) -> spannungsgrenze/1
  [Lm] -> MTPC-Kennlinie/3(Lm)
  [p] -> MTPF-Kennlinie/13(p)
  ID/1 -> " Vorberechnung gemeinsamer Größen"/1(ID), [ID]
  [IQ] -> MTPC-Kennlinie/7(IQ)
  [ID] -> MTPC-Kennlinie/6(ID)
  [IQ] -> MTPF-Kennlinie/15(IQ)
  [Lq2] -> MTPF-Kennlinie/7(Lq2)
  " Vorberechnung gemeinsamer Größen"/12(stromgrenze) -> stromgrenze/1
  " Vorberechnung gemeinsamer Größen"/5(Ld2) -> [Ld2]
  [Ld_q] -> MTPF-Kennlinie/8(Ld_q)
  [Lm] -> MTPF-Kennlinie/1(Lm)
  [PSID] -> MTPF-Kennlinie/11(PSID)
  " Vorberechnung gemeinsamer Größen"/11(Rs2) -> [Rs2]
  [Ld] -> MTPV-Kennlinie/2(Ld)
  " Vorberechnung gemeinsamer Größen"/6(Lq2) -> [Lq2]
  [Lq] -> MTPF-Kennlinie/3(Lq)
  [Lm2] -> MTPF-Kennlinie/10(Lm2)
  [Lq_d] -> MTPF-Kennlinie/9(Lq_d)
  [Ld2] -> MTPV-Kennlinie/5(Ld2)
  [p] -> MTPV-Kennlinie/12(p)
  " Vorberechnung gemeinsamer Größen"/9(psiq1) -> [psiq1]
  [Lm2] -> MTPV-Kennlinie/4(Lm2)
  [PSIQ] -> MTPV-Kennlinie/11(PSIQ)
  " Vorberechnung gemeinsamer Größen"/2(Ldq_p) -> [Ldq_p]
  [Ldq] -> MTPC-Kennlinie/4(Ldq)
  [psiq1] -> MTPC-Kennlinie/2(psiq1)
  [psid1] -> MTPC-Kennlinie/1(psid1)

== matlab function Model_Linearisierung_final/Subsystem Arbeitspunktsteuerung/Arbeitspunktsteuerung/Iterationsblock ==
  data: start_cmd input; id_iter output; id0 input; iq0 input; id_soll input; iq_soll input; I_max input; iq_iter output; id_final output; iq_final output; iter_count output; status_flag output; delta_id output; delta_iq output
function [id_iter, iq_iter, id_final, iq_final, ...
          iter_count, status_flag, delta_id, delta_iq] = ...
    fcn(start_cmd, id0, iq0, ...
        id_soll, iq_soll, I_max)

% Eingang: Startsignal, Startarbeitspunkt (idq_init), Sollarbeitspunkt aus
% Schätzung (idq_soll), Strombegrenzung, Strategie
% Ausgang: aktueller Iterationspunkt (idq_iter), finale Arbeitspunkt
% (idq_final), Flag für beendete Iteration, gültige Lösung, Zähler
% Iterationen

%#codegen

%% Legende Strategiewahl:
%   0 = Fehler / kein gültiger Arbeitspunkt
%   1 = i_ac = MTPC ∩ Stromgrenze
%   2 = i_vv = MTPV ∩ Spannungsellipse
%   3 = i_av = MTPC ∩ Spannungsellipse
%   4 = i_cv = Stromgrenze ∩ Spannungsellipse
%   5 = i_at = MTPC ∩ Drehmoment
%   6 = i_tv = Spannungsellipse ∩ Drehmoment
% ---------------------------------------------------------

% Parameter
I_nenn = I_max;  % Setze Nennstrom auf angenommenen Maximalstrom
lambda  = 0.5;   % Dämpfungsfator Iterationen (Annahme aus Masterarbeit Köster)
maxIter = uint16(50);    % maximale Anzahl der Iterationen bis Abbruch, vorerst 20, ggf 10?  uint16(20)
eps_i   = 0.02*I_nenn;   % Abbruch bei Fehler < 2% des Nennstroms
strategy_in= uint8(0);
delta_id = 0.0;
delta_iq = 0.0;

% Persistent Variablen: (= Zustandsautomat)
% aktuelle Iterationszustand wird zwischen den Funktionsaufrufen gespeichert
persistent id_state
persistent iq_state

persistent k_state

persistent active_state
persistent done_state
persistent valid_state

persistent strategy_state

persistent start_old

% Initialisierung der Variablen bei ersten Funktionsaufruf
if isempty(id_state)
    % Initialisierung Ausgänge
    id_iter = 0.0;
    iq_iter = 0.0;
    id_final = 0.0;
    iq_final = 0.0;
    id_state = 0.0;
    iq_state = 0.0;
    k_state = uint16(0);
    active_state = false;
    done_state   = false;
    strategy_state = uint8(0);
    %status_flag    = uint8(0);
    valid_state = false;
    start_old = false;
end

% ---------------------------------------------------------
%  NaN & Inf Check für Sollwerte aus Glac
% ---------------------------------------------------------
if isnan(id_soll) || isnan(iq_soll) || isinf(id_soll) || isinf(iq_soll)
    % Notbremse: Glac hat keine Lösung gefunden. 
    % Abbrechen der Iteration für diesen Zyklus 
    valid_state  = false;
    done_state   = true;
    active_state = false;
    status_flag  = uint8(3); % Fehler / Ungültig
    
    id_iter = id_state; % Letzten gültigen Zustand beibehalten
    iq_iter = iq_state;
    id_final = 0;
    iq_final = 0;
    iter_done = done_state;
    iter_valid = valid_state;
    iter_count = double(k_state);
    strategy_out = strategy_state;
    return;
end

% ---------------------------------------------------------
% Start einer neuen Iteration nur auf positiver Flanke
% ---------------------------------------------------------
% start_rise = start_cmd && ~start_old;
% start_old = start_cmd;      

if start_cmd
    id_state = id0;     % Startpunkt für neue Iteration
    iq_state = iq0;
    k_state  = uint16(0);
    active_state = true;
    done_state   = false;
    valid_state  = false;
    strategy_state = uint8(0);
    
end

% ---------------------------------------------------------
% Falls nicht aktiv: nur aktuellen Zustand ausgeben
% ---------------------------------------------------------
if ~active_state
    id_iter = id_state;
    iq_iter = iq_state;
    id_final = id_state;
    iq_final = iq_state;
    iter_done = done_state;
    iter_valid = valid_state;
    iter_count = double(k_state);
    strategy_out = strategy_state;
    if done_state
        if valid_state
            status_flag = uint8(2);
        else
            status_flag = uint8(3);
        end
    else
        status_flag = uint8(0);
    end
    return;
end

% ---------------------------------------------------------
% Fehlernorm - Berechnung Fehler zwischen aktuellem und gewünschtem
% Arbeitspunkt
% ---------------------------------------------------------
err_d = id_soll - id_state;     % Abweichung Strom id
err_q = iq_soll - iq_state;     % Abweichung Strom iq
err_norm = sqrt(err_d*err_d + err_q*err_q); % Normierter Fehler der Ströme

% ---------------------------------------------------------
% Konvergenz -
% nur wenn Stromvektorfehler klein genug
% ---------------------------------------------------------
if err_norm <= eps_i
    id_state = id_soll;     % Setze id_state = id_soll
    iq_state = iq_soll;     % Setze iq_state = iq_soll
    strategy_state = strategy_in;
    valid_state  = true;
    done_state   = true;
    active_state = false;   % Iteration nicht mehr aktiv

    id_iter = id_state; 
    iq_iter = iq_state;
    id_final = id_state;
    iq_final = iq_state;
    iter_done  = true;
    iter_valid = true;
    iter_count = double(k_state);
    strategy_out = strategy_state;
    status_flag = uint8(2);
    return;
end

% ---------------------------------------------------------
% Falls keine Konvergenz (Abweichung <2% I_nenn) erreicht wird: 
% Abbruch der Iteration
% ---------------------------------------------------------
if k_state >= maxIter
    valid_state  = false;
    done_state   = true;
    active_state = false;
    strategy_state = strategy_in;

    id_iter = id_state;
    iq_iter = iq_state;
    id_final = 0;
    iq_final = 0;
    iter_done = true;
    iter_valid = false;
    iter_count = double(k_state);
    strategy_out = strategy_state;
    status_flag = uint8(3); % Flag 3: Ungültige Lösung
    return;
end

% ---------------------------------------------------------
% Gedämpftes Update: 
% idq_k+1 = idq_k + lamda*(idq_soll-idq_k)
% lamda = 0.5: Fehler wird pro Schritt halbiert, 
% neuer AP liegt zwischen altem und gewünschtem Wert
% Schrittweitenbegrenzung
% ---------------------------------------------------------
id_state = id_state + lambda * err_d;
iq_state = iq_state + lambda * err_q;
k_state = k_state + uint16(1);  % Iterationszähler hochzählen
strategy_state = strategy_in;

% Delta Werte für Linearisierung:
delta_id = lambda * err_d;
delta_iq = lambda * err_q;

id_iter = id_state;
iq_iter = iq_state;
id_final = 0; % id_state;
iq_final = 0; % iq_state;
iter_done  = false;          % Iter_done = false: Weitere Iterationen nötig
iter_valid = false;
iter_count = double(k_state);
strategy_out = strategy_state;
status_flag = uint8(1);     % Statusflag = 1: Laufender Iterationsprozess
end

== matlab function Model_Linearisierung_final/Subsystem Arbeitspunktsteuerung/Arbeitspunktsteuerung/Startflanke für Berechnung ==
  data: T_soll input; start_cmd output; omega input; T_soll_z1 input; omega_z1 input
function start_cmd  = ...
    fcn(T_soll, omega, T_soll_z1, omega_z1)

dT = abs(T_soll - T_soll_z1);   % Änderung Drehmoment
dOmega = abs(omega - omega_z1); % Änderung Drehzahl

if dT > 0 || dOmega > 0
    start_cmd = true;
else
    start_cmd = false;
end

== matlab function Model_Linearisierung_final/Subsystem Arbeitspunktsteuerung/Arbeitspunktsteuerung/Glac - Arbeitspunktwahl ==
  data: i_ac input; i_vv input; i_av input; i_cv input; i_at input; i_tv input; psi_bar_d input; psi_bar_q input; Ldd input; Lqq input; Ldq input; Lqd input; Imax input; Umax input; Rs input; omega input; p input; T_soll input; id_soll output; iq_soll output; strategy_flag output
function [id_soll, iq_soll, strategy_flag] = ...
    Arbeitspunktwahl_Glac(i_ac, i_vv, i_av, i_cv, i_at, i_tv, ...
            psi_bar_d, psi_bar_q, Ldd, Lqq, Ldq, Lqd, ...
            Imax, Umax, Rs, omega, p, T_soll)

%#codegen
coder.extrinsic('disp');
% ================================================================
% ARBEITSPUNKTWAHL NACH GLAC
%
% Eingänge:
%   i_ac  : MTPC ∩ Stromkreis
%   i_vv  : MTPV ∩ Spannungskurve
%   i_av  : MTPC ∩ Spannungskurve
%   i_cv  : Stromkreis ∩ Spannungskurve
%   i_at  : MTPC ∩ Drehmomentkurve
%   i_tv  : Spannungskurve ∩ Drehmomentkurve
%
% Die Schnittpunkte werden vom vorhergehenden Block bereits
% nach Glac sortiert:
%
%   Zeile 1 = kleinste gewichtete Norm
%   Zeile 2 = zweitkleinste
%   Zeile 3 = drittkleinste
%   Zeile 4 = größte gewichtete Norm
%
% Jeder Eingang ist 4x2:
%   [id1 iq1
%    id2 iq2
%    id3 iq3
%    id4 iq4]
%
% Block 4 wählt daraus den physikalisch relevanten Punkt.
%
% strategy_flag:
%   0 = Fehler
%   1 = i_ac
%   2 = i_vv
%   3 = i_av
%   4 = i_cv
%   5 = i_at
%   6 = i_tv
% ================================================================

    %% 0. Initialisierung
    id_soll = 0;
    iq_soll = 0;
    strategy_flag = uint8(0);

    % Initialisierung relativer Toleranzen 
    tol_I  = Imax * 1.001; 
    tol_U2 = Umax^2 * 1.002;

   %% 2. Relevanten Kandidaten aus den 4x2-Matrizen auswählen LM PRÜFEN ???
    % Es wird der erste physikalisch passende Kandidat gewählt.
    % Die Reihenfolge stammt aus der Glac-Sortierung in Block 3.
    %
    % Zusätzlich wird bei den nicht direkt drehmomentdefinierten
    % Schnittpunkten auf das Vorzeichen des gewünschten Drehmoments geachtet.

    i_ac_sel = selectPoint(i_ac, T_soll, psi_bar_d, psi_bar_q, Ldd, Lqq, Ldq, Lqd, p);
    
    i_vv_sel = selectPoint(i_vv, T_soll, psi_bar_d, psi_bar_q, Ldd, Lqq, Ldq, Lqd, p);
    
    i_av_sel = selectPoint(i_av, T_soll, psi_bar_d, psi_bar_q, Ldd, Lqq, Ldq, Lqd, p);
    
    i_cv_sel = selectPoint(i_cv, T_soll, psi_bar_d, psi_bar_q, Ldd, Lqq, Ldq, Lqd, p);
    
    i_at_sel = selectPoint(i_at, T_soll, psi_bar_d, psi_bar_q, Ldd, Lqq, Ldq, Lqd, p);
    
    i_tv_sel = selectPoint(i_tv, T_soll, psi_bar_d, psi_bar_q, Ldd, Lqq, Ldq, Lqd, p);

    %% 3. Zulässigen Grenzpunkt bestimmen
    i_feas = [NaN NaN];
    feas_tag = uint8(0);    
   
    % FALL 1: i_vv existiert und liegt innerhalb des Stromkreises
    if isFinitePoint(i_vv_sel)
        I_vv = hypot(i_vv_sel(1), i_vv_sel(2));
    
        if I_vv <= tol_I
            i_feas = i_vv_sel;
            feas_tag = uint8(2);
    
        else
            % i_vv liegt außerhalb des Stromkreises.
            % Vergleich psi_cv und psi_ac.
            psi_ac = NaN;
            psi_cv = NaN;
    
            if isFinitePoint(i_ac_sel)
                psi_ac = fluxSquared(i_ac_sel(1), i_ac_sel(2), ...
                    psi_bar_d, psi_bar_q, Ldd, Lqq, Ldq, Lqd);
            end
    
            if isFinitePoint(i_cv_sel)
                psi_cv = fluxSquared(i_cv_sel(1), i_cv_sel(2), ...
                    psi_bar_d, psi_bar_q, Ldd, Lqq, Ldq, Lqd);  
            end
    
            if isfinite(psi_ac) && isfinite(psi_cv)    
                if psi_cv > psi_ac    
                    i_feas = i_ac_sel;
                    feas_tag = uint8(1);
    
                else   
                    i_feas = i_cv_sel;
                    feas_tag = uint8(4);  
                end
    
            elseif isFinitePoint(i_ac_sel)   
                i_feas = i_ac_sel;
                feas_tag = uint8(1);
    
            elseif isFinitePoint(i_cv_sel)    
                i_feas = i_cv_sel;
                feas_tag = uint8(4);  
            end
        end
    end
        
    % FALL 2: i_vv existiert nicht    
    if ~isFinitePoint(i_feas)    
        if isFinitePoint(i_ac_sel)   
            i_feas = i_ac_sel;
            feas_tag = uint8(1);
    
        elseif isFinitePoint(i_cv_sel)    
            i_feas = i_cv_sel;
            feas_tag = uint8(4);
    
        elseif isFinitePoint(i_tv_sel)    
            i_feas = i_tv_sel;
            feas_tag = uint8(6);    
        end
    end
       
    %% 4. Maximales verfügbares Drehmoment
    m_max = NaN;
   
    if isFinitePoint(i_feas)    
        m_max = torqueAtPoint(i_feas(1), i_feas(2), psi_bar_d, psi_bar_q, Ldd, Lqq, Ldq, Lqd, p);    
    end
    
    
    %% 5. Drehmoment am MTPC-Spannungsschnittpunkt
    m_av = NaN;
    
    if isFinitePoint(i_av_sel)    
        I_av = hypot(i_av_sel(1), i_av_sel(2));    
        U2_av = voltageSquared(i_av_sel(1), i_av_sel(2), ...
            psi_bar_d, psi_bar_q, Ldd, Lqq, Ldq, Lqd, Rs, omega);
    
        if I_av <= tol_I && U2_av <= Umax^2 * 1.002    
            m_av = torqueAtPoint(i_av_sel(1), i_av_sel(2), ...
                psi_bar_d, psi_bar_q, Ldd, Lqq, Ldq, Lqd, p);  
        end
    end
    
    
    % Falls kein gültiger MTPC-Spannungsschnittpunkt vorhanden ist   
    if ~isfinite(m_av) && isfinite(m_max)  
        m_av = m_max;   
    end
    
    % MTPC-Bereich darf nicht größer als das maximal verfügbare
    % Drehmoment sein
    if isfinite(m_av) && isfinite(m_max)    
        if abs(m_av) > abs(m_max)   
            m_av = m_max;  
        end
    end
    
    
    %% 6. Arbeitspunktwahl
    % FALL 1:
    % Sollmoment innerhalb des MTPC-Bereichs    
    if isfinite(m_av)
    
        if abs(T_soll) <= abs(m_av)
    
            if isFinitePoint(i_at_sel)    
                I_at = hypot(i_at_sel(1), i_at_sel(2));
                U2_at = voltageSquared(i_at_sel(1), i_at_sel(2), ...
                    psi_bar_d, psi_bar_q, Ldd, Lqq, Ldq, Lqd, Rs, omega);
    
                if I_at <= tol_I && U2_at <= Umax^2 * 1.002   
                    id_soll = i_at_sel(1);
                    iq_soll = i_at_sel(2);
    
                    strategy_flag = uint8(5);
    
                    return;   
                end
            end
        end
    end
    
    % FALL 2:
    % Sollmoment unterhalb des maximal verfügbaren Moments
    % -> Spannung begrenzt    
    if isfinite(m_max)
        
        if abs(T_soll) <= abs(m_max)
    
            if isFinitePoint(i_tv_sel)
    
                I_tv = hypot(i_tv_sel(1), i_tv_sel(2));    
                U2_tv = voltageSquared(i_tv_sel(1), i_tv_sel(2), ...
                    psi_bar_d, psi_bar_q, Ldd, Lqq, Ldq, Lqd, Rs, omega);
    
                if I_tv <= tol_I && U2_tv <= Umax^2 * 1.002   
                    id_soll = i_tv_sel(1);
                    iq_soll = i_tv_sel(2);
    
                    strategy_flag = uint8(6);
    
                    return;    
                end
            end
        end
    end
    
    
    %% 7. Sollmoment nicht erreichbar
    % -> maximal zulässiger Grenzpunkt    
    if isFinitePoint(i_feas)    
        I_feas = hypot(i_feas(1), i_feas(2));    
        U2_feas = voltageSquared(i_feas(1), i_feas(2), ...
            psi_bar_d, psi_bar_q, Ldd, Lqq, Ldq, Lqd, Rs, omega);
    
        if I_feas <= tol_I && U2_feas <= Umax^2 * 1.002    
            id_soll = i_feas(1);
            iq_soll = i_feas(2);
    
            strategy_flag = feas_tag;
    
            return;    
        end
    end


%%%%%%%%%%%%%%%%%%%%%%%%%%%%%%%%%%%%%%%%%%%%%%%%%%%%%%%%%%%%%%%%%%%%%%%%%    
    function p_sel = selectPoint(P, Tref, psi_bar_d, psi_bar_q, ...
                             Ldd, Lqq, Ldq, Lqd, p)

    p_sel = [NaN NaN];

    for k = 1:4

        id = P(k,1);
        iq = P(k,2);

        if isfinite(id) && isfinite(iq)

            T = torqueAtPoint(id, iq, psi_bar_d, psi_bar_q, Ldd, Lqq, Ldq, Lqd, p);
            % Für T_soll ~= 0 muss das Drehmomentvorzeichen
            % zum gewünschten Drehmoment passen.

            if abs(Tref) > 1e-6
                % 1. Drehmomentvorzeichen muss zum Sollmoment passen
                if sign(T) ~= sign(Tref)  % Wenn Vorzeichen T und Tref ungleich
                    continue;             % Punkt verwerfen
                end

                 % 2. iq muss zwingend dasselbe Vorzeichen wie Tref haben 
                if (Tref > 0 && iq < 0) || (Tref < 0 && iq > 0) % Wenn Vorzeichen ungleich
                    continue;                                   % Punkt verwerfen
                end
                
                 % 3. Beschränkung auf den gültigen Kennfeldbereich (2. Quadrant: id <= 0)
                if id > 0           % Wen id >0
                    continue;       % Punkt verwerfen
                end
            end

            p_sel = [id iq];
            return;

        end
    end

end


function tf = isFinitePoint(P)

    tf = numel(P) == 2 && isfinite(P(1)) && isfinite(P(2));

end


function psi2 = fluxSquared(id, iq, psi_bar_d, psi_bar_q, Ldd, Lqq, Ldq, Lqd)

    psi_d = psi_bar_d + Ldd * id + Ldq * iq;
    psi_q = psi_bar_q + Lqd * id + Lqq * iq;

    psi2 = psi_d^2 + psi_q^2;

end


function T = torqueAtPoint(id, iq, psi_bar_d, psi_bar_q, Ldd, Lqq, Ldq, Lqd, p)

    psi_d = psi_bar_d + Ldd * id + Ldq * iq;
    psi_q = psi_bar_q + Lqd * id + Lqq * iq;

    T = 1.5 * p * (psi_d * iq - psi_q * id);

end


function U2 = voltageSquared(id, iq, psi_bar_d, psi_bar_q, Ldd, Lqq, Ldq, Lqd, Rs, omega)

    psi_d = psi_bar_d + Ldd * id + Ldq * iq;
    psi_q = psi_bar_q + Lqd * id + Lqq * iq;

    ud = Rs * id - omega * psi_q;
    uq = Rs * iq + omega * psi_d;

    U2 = ud^2 + uq^2;

end

end
